simulink model "One_compartment_linear_thorax"  (R2019b)
settings: Solver=VariableStepAuto  StartTime=0.0  StopTime=50  FixedStep=0.01  RelTol=1e-3
values from neighbouring files (symbols this model uses):
  breath = 60/f    (= 4)    [Model_simulation.m]
  E1 = 10    [Model_simulation.m]
  E_th = 15    [Model_simulation.m]
  insptime = (ieratio(1)/(ieratio(1)+ieratio(2)))*100    [Model_simulation.m]
  Pcontrol = 5    [Model_simulation.m]
  PEEP = 5    [Model_simulation.m]
  R1 = 5    [Model_simulation.m]
  V0 = 2    [Model_simulation.m]
  V0_th = 4.6    [Model_simulation.m]
settings Model: Creator=Amne  LastModifiedBy=Amne
settings DataIOCC: ReturnWorkspaceOutputsName=SDOSimTest_Log
settings DebuggingCC: ArithmeticOperatorsInVariantConditions=warning
settings SFSimCC: SimUseLocalCustomCode=off  CustomCodeUndefinedFunction=UseInterfaceOnly
settings RTWCC: RTWUseLocalCustomCode=off

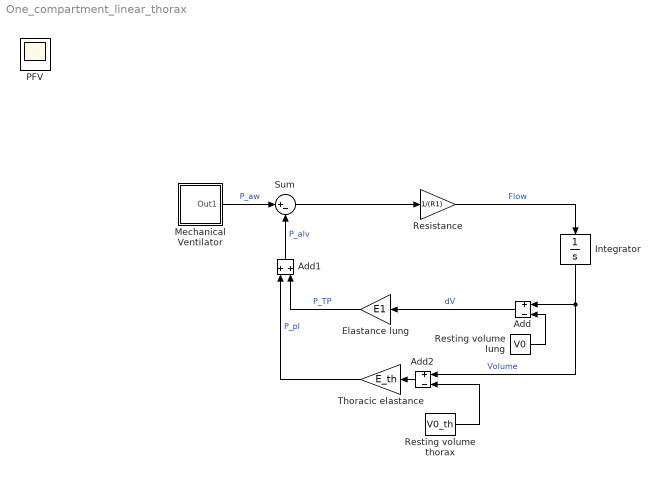
== system One_compartment_linear_thorax ==
  Add : Sum  Inputs=+-
  Add1 : Sum
  Add2 : Sum  Inputs=+-
  Elastance lung : Gain  Gain=E1
  Integrator : Integrator  ZeroCross=off
  "Mechanical Ventilator " : Subsystem
  Resistance : Gain  Gain=1/(R1)
  Resting volume lung : Constant  Value=V0
  Resting volume thorax : Constant  Value=V0_th
  Sum : Sum  Inputs=|+-
  Thoracic elastance : Gain  Gain=E_th
  PFV : Scope
  wires:
  Integrator/1 -> Add/1, Add2/1  "Volume"
  Elastance lung/1 -> Add1/2  "P_TP"
  Resistance/1 -> Integrator/1  "Flow"
  Sum/1 -> Resistance/1
  Add/1 -> Elastance lung/1  "dV"
  Resting volume lung/1 -> Add/2
  "Mechanical Ventilator "/1(Out1) -> Sum/1  "P_aw"
  Thoracic elastance/1 -> Add1/1  "P_pl"
  Add1/1 -> Sum/2  "P_alv"
  Resting volume thorax/1 -> Add2/2
  Add2/1 -> Thoracic elastance/1

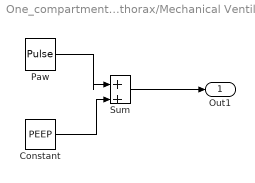
== system One_compartment_linear_thorax/Mechanical Ventilator  ==
  Constant : Constant  Value=PEEP  SampleTime=0.1
  Paw : DiscretePulseGenerator  PulseType=Time based  Amplitude=Pcontrol  Period=breath  PulseWidth=insptime  PhaseDelay=2  SampleTime=0.1
  Sum : Sum  Inputs=|++
  Out1 : Outport  VectorParamsAs1DForOutWhenUnconnected=off
  wires:
  Paw/1 -> Sum/1
  Constant/1 -> Sum/2
  Sum/1 -> Out1/1
